simulink model "sys_kucukay"  (R2021b)
settings: Solver=VariableStepAuto  StartTime=0.0  StopTime=10.0  RelTol=1e-3
undefined symbols (not defined in the file): cog_height, DiscIntNeverNeededParam, g, lF, pitch_inertia, r, sprung_mass
settings Model: Creator=I012488  LastModifiedBy=I012488

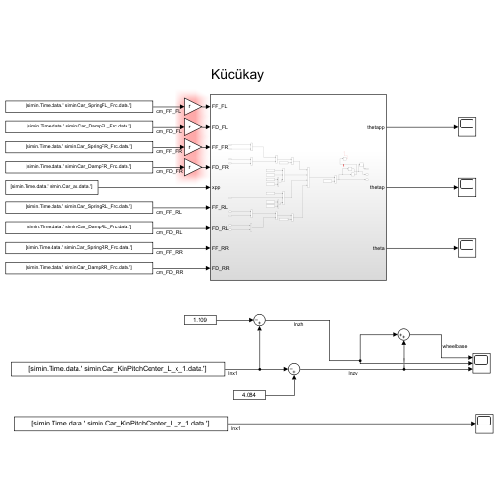
[thumbnail: Simulink's stored preview of the top-level diagram]
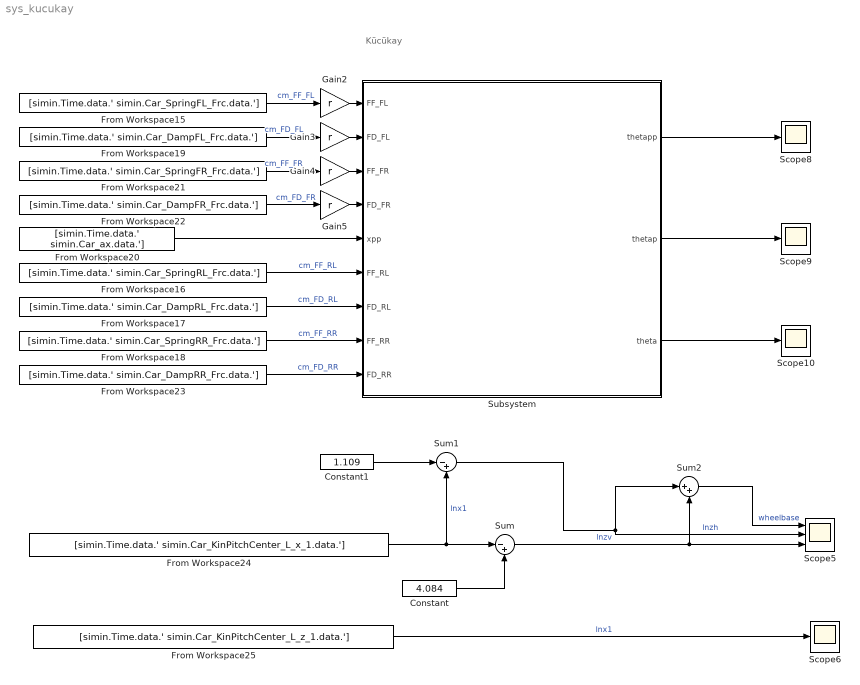
== system sys_kucukay ==
  note: Kücükay
  Constant : Constant  Value=4.084
  Constant1 : Constant  Value=1.109
  From Workspace15 : FromWorkspace  VariableName=[simin.Time.data.' simin.Car_SpringFL_Frc.data.']
  From Workspace16 : FromWorkspace  VariableName=[simin.Time.data.' simin.Car_SpringRL_Frc.data.']
  From Workspace17 : FromWorkspace  VariableName=[simin.Time.data.' simin.Car_DampRL_Frc.data.']
  From Workspace18 : FromWorkspace  VariableName=[simin.Time.data.' simin.Car_SpringRR_Frc.data.']
  From Workspace19 : FromWorkspace  VariableName=[simin.Time.data.' simin.Car_DampFL_Frc.data.']
  From Workspace20 : FromWorkspace  VariableName=[simin.Time.data.' simin.Car_ax.data.']
  From Workspace21 : FromWorkspace  VariableName=[simin.Time.data.' simin.Car_SpringFR_Frc.data.']
  From Workspace22 : FromWorkspace  VariableName=[simin.Time.data.' simin.Car_DampFR_Frc.data.']
  From Workspace23 : FromWorkspace  VariableName=[simin.Time.data.' simin.Car_DampRR_Frc.data.']
  From Workspace24 : FromWorkspace  VariableName=[simin.Time.data.' simin.Car_KinPitchCenter_L_x_1.data.']
  From Workspace25 : FromWorkspace  VariableName=[simin.Time.data.' simin.Car_KinPitchCenter_L_z_1.data.']
  Gain{2..5} (4 alike) : Gain  Gain=r
  Scope{6,8..10} (4 alike) : Scope
  Scope5 : Scope  NumInputPorts=3
  Subsystem : Subsystem
  Sum : Sum  Inputs=|-+
  Sum1 : Sum  Inputs=|-+
  Sum2 : Sum  Inputs=|++
  wires:
  Sum1/1 -> Sum2/1, Scope5/2  "lnzh"
  Gain4/1 -> Subsystem/3(FF_FR)
  Subsystem/2(thetap) -> Scope9/1
  From Workspace22/1 -> Gain5/1  "cm_FD_FR"
  Subsystem/1(thetapp) -> Scope8/1
  Sum2/1 -> Scope5/1  "wheelbase"
  Gain2/1 -> Subsystem/1(FF_FL)
  Subsystem/3(theta) -> Scope10/1
  From Workspace25/1 -> Scope6/1  "lnx1"
  Constant1/1 -> Sum1/1
  Gain3/1 -> Subsystem/2(FD_FL)
  From Workspace17/1 -> Subsystem/7(FD_RL)  "cm_FD_RL"
  From Workspace18/1 -> Subsystem/8(FF_RR)  "cm_FF_RR"
  From Workspace23/1 -> Subsystem/9(FD_RR)  "cm_FD_RR"
  Constant/1 -> Sum/2
  From Workspace15/1 -> Gain2/1  "cm_FF_FL"
  From Workspace21/1 -> Gain4/1  "cm_FF_FR"
  From Workspace16/1 -> Subsystem/6(FF_RL)  "cm_FF_RL"
  From Workspace24/1 -> Sum/1, Sum1/2  "lnx1"
  Gain5/1 -> Subsystem/4(FD_FR)
  Sum/1 -> Sum2/2, Scope5/3  "lnzv"
  From Workspace20/1 -> Subsystem/5(xpp)
  From Workspace19/1 -> Gain3/1  "cm_FD_FL"

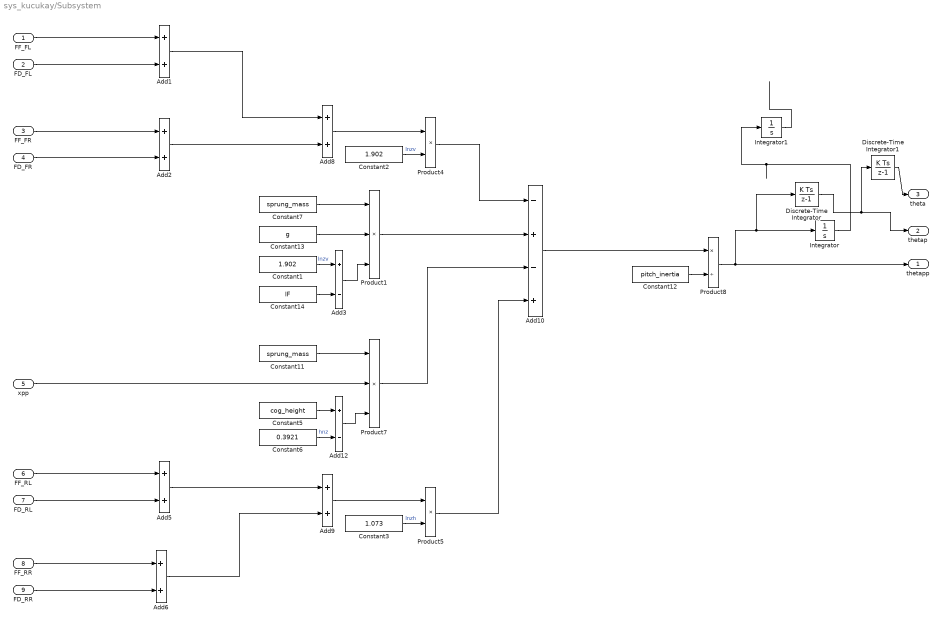
== system sys_kucukay/Subsystem ==
  FF_FL : Inport
  FD_FL : Inport  Port=2
  FF_FR : Inport  Port=3
  FD_FR : Inport  Port=4
  xpp : Inport  Port=5
  FF_RL : Inport  Port=6
  FD_RL : Inport  Port=7
  FF_RR : Inport  Port=8
  FD_RR : Inport  Port=9
  Add{1..2,5..6,8..9} (6 alike) : Sum
  Add10 : Sum  Inputs=-+-+
  Add12 : Sum  Inputs=+-
  Add3 : Sum  Inputs=+-
  Constant1 : Constant  Value=1.902
  Constant11 : Constant  Value=sprung_mass
  Constant12 : Constant  Value=pitch_inertia
  Constant13 : Constant  Value=g
  Constant14 : Constant  Value=lF
  Constant2 : Constant  Value=1.902  VectorParams1D=off
  Constant3 : Constant  Value=1.073
  Constant5 : Constant  Value=cog_height
  Constant6 : Constant  Value=0.3921
  Constant7 : Constant  Value=sprung_mass
  Discrete-Time Integrator : DiscreteIntegrator  SampleTime=0.01  ICPrevOutput=DiscIntNeverNeededParam  ICPrevScaledInput=DiscIntNeverNeededParam
  Discrete-Time Integrator1 : DiscreteIntegrator  InitialCondition=-0.001  SampleTime=0.01  ICPrevOutput=DiscIntNeverNeededParam  ICPrevScaledInput=DiscIntNeverNeededParam
  Integrator : Integrator
  Integrator1 : Integrator  InitialCondition=1.439e-07
  Product1 : Product  Inputs=3  RndMeth=Zero
  Product4 : Product  RndMeth=Zero
  Product5 : Product  RndMeth=Zero
  Product7 : Product  Inputs=3  RndMeth=Zero
  Product8 : Product  Inputs=*/  RndMeth=Zero
  thetapp : Outport
  thetap : Outport  Port=2
  theta : Outport  Port=3
  wires:
  Add8/1 -> Product4/1
  FD_FR/1 -> Add2/2
  Add2/1 -> Add8/2
  Constant2/1 -> Product4/2  "lnzv"
  Product4/1 -> Add10/1
  Add1/1 -> Add8/1
  FF_FR/1 -> Add2/1
  FF_FL/1 -> Add1/1
  FD_FL/1 -> Add1/2
  Product1/1 -> Add10/2
  Constant14/1 -> Add3/2
  Constant13/1 -> Product1/2
  Constant1/1 -> Add3/1  "lnzv"
  Constant7/1 -> Product1/1
  Add3/1 -> Product1/3
  Constant5/1 -> Add12/1
  Add12/1 -> Product7/3
  Constant6/1 -> Add12/2  "hnz"
  xpp/1 -> Product7/2
  Constant11/1 -> Product7/1
  Product7/1 -> Add10/3
  FD_RL/1 -> Add5/2
  FD_RR/1 -> Add6/2
  Add6/1 -> Add9/2
  Add5/1 -> Add9/1
  Add9/1 -> Product5/1
  Constant3/1 -> Product5/2  "lnzh"
  FF_RL/1 -> Add5/1
  FF_RR/1 -> Add6/1
  Product5/1 -> Add10/4
  Product8/1 -> Discrete-Time Integrator/1, Integrator/1, thetapp/1
  Add10/1 -> Product8/1
  Integrator1/1 -> ?
  Constant12/1 -> Product8/2
  Integrator/1 -> Integrator1/1
  Discrete-Time Integrator/1 -> thetap/1, Discrete-Time Integrator1/1
  Discrete-Time Integrator1/1 -> theta/1
